simulink model "DPLL"  (R2013a)
settings: Solver=ode45  StartTime=0.0  StopTime=12000/1200  RelTol=1e-3
undefined symbols (not defined in the file): DiscIntNeverNeededParam
libraries: dspsigops x4, commfilt2 x3, dsparch4 x3, commsynccomp2 x2, commchan3 x1, commsink2 x1, commrandsrc2 x1
settings Model: Creator=Cedric  LastModifiedBy=Cedric

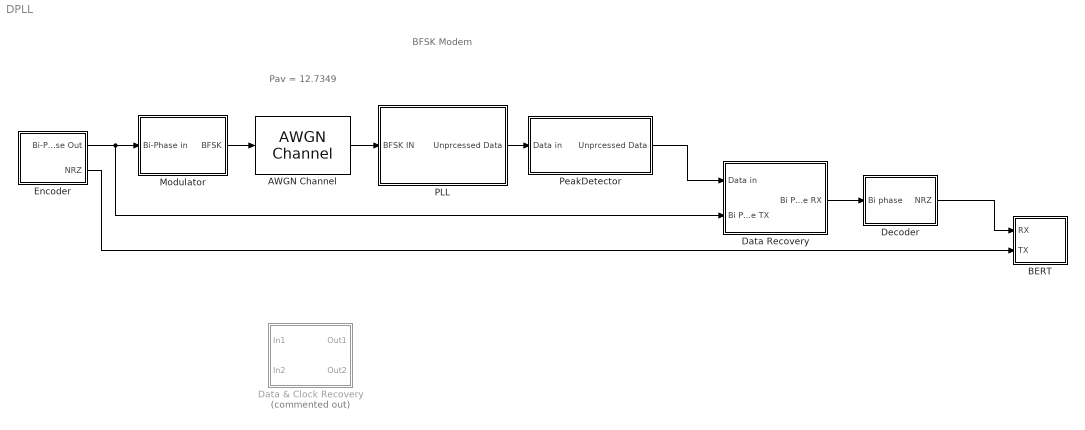
== system DPLL ==
  note: BFSK Modem
  note: Pav = 12.7349
  AWGN Channel : commchan3/AWGN Channel  InputProcessing=Columns as channels (frame based)  seed=randseed  noiseMode="Signal to noise ratio  (SNR)"  EbNodB=10  EsNodB=10  SNRdB=1000  bitsPerSym=1  Ps=12.7349  Tsym=1  variance=5
  BERT : Subsystem
  Data & Clock Recovery : Subsystem  Commented=on
  Data Recovery : Subsystem
  Decoder : Subsystem
  Encoder : Subsystem
  Modulator : Subsystem
  PLL : Subsystem
  PeakDetector : Subsystem
  wires:
  Modulator/1(BFSK) -> AWGN Channel/1
  Decoder/1(NRZ) -> BERT/1(RX)
  AWGN Channel/1 -> PLL/1(BFSK IN)
  Encoder/2(NRZ) -> BERT/2("TX ")
  PLL/1(Unprcessed Data) -> PeakDetector/1(Data in)
  Encoder/1(Bi-Phase Out) -> Data Recovery/2(Bi Phase TX), Modulator/1(Bi-Phase in)
  PeakDetector/1(Unprcessed Data) -> Data Recovery/1(Data in)
  Data Recovery/1(Bi Phase RX) -> Decoder/1(Bi phase)

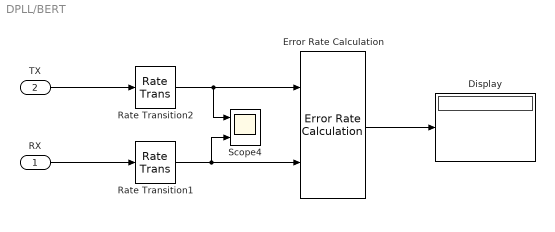
== system DPLL/BERT ==
  RX : Inport
  "TX " : Inport  Port=2
  Display : Display
  Error Rate Calculation : commsink2/Error Rate Calculation  N=1  st_delay=0  cp_mode=Entire frame  subframe=[]  PMode=Port  WsName=ErrorVec  RsMode2=off  stop=off  numErr=100  maxBits=1e6
  Rate Transition1 : RateTransition  OutPortSampleTime=1/(1200)
  Rate Transition2 : RateTransition  OutPortSampleTime=1/(1200)
  Scope4 : Scope  NumInputPorts=2
      settings: YMin=47500~-0.5  YMax=90000~1.5  SaveName=ScopeData3
  wires:
  Error Rate Calculation/1 -> Display/1
  "TX "/1 -> Rate Transition2/1
  RX/1 -> Rate Transition1/1
  Rate Transition1/1 -> Scope4/2, Error Rate Calculation/2
  Rate Transition2/1 -> Scope4/1, Error Rate Calculation/1

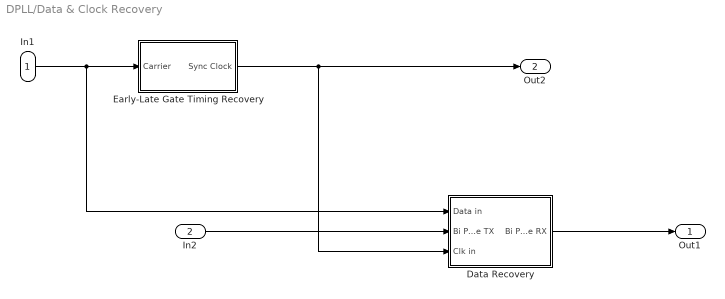
== system DPLL/Data & Clock Recovery ==
  In1 : Inport
  In2 : Inport  Port=2
  Data Recovery : Subsystem
  Early-Late Gate Timing Recovery : Subsystem
  Out1 : Outport
  Out2 : Outport  Port=2
  wires:
  Data Recovery/1(Bi Phase RX) -> Out1/1
  In2/1 -> Data Recovery/2(Bi Phase TX)
  Early-Late Gate Timing Recovery/1(Sync Clock) -> Data Recovery/3(Clk in), Out2/1
  In1/1 -> Early-Late Gate Timing Recovery/1(Carrier), Data Recovery/1(Data in)

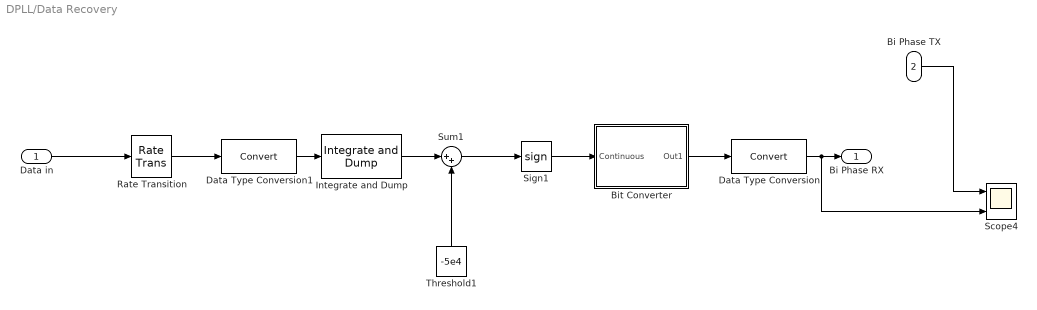
== system DPLL/Data Recovery ==
  Data in : Inport
  Bi Phase TX : Inport  Port=2
  Bit Converter : Subsystem
  Data Type Conversion : DataTypeConversion
  Data Type Conversion1 : DataTypeConversion
  Integrate and Dump : commfilt2/Integrate and Dump  obssamples=1024  offsetsamples=0  nodump=off  roundingMode=Floor  overflowMode=off
  Rate Transition : RateTransition  OutPortSampleTime=1/(1200*1024)
  Scope4 : Scope  NumInputPorts=2
      settings: YMin=47500~-0.5  YMax=90000~1.5  SaveName=ScopeData8
  Sign1 : Signum
  Sum1 : Sum  Inputs=|++
  Threshold1 : Constant  Value=-5e4
  Bi Phase RX : Outport
  wires:
  Data in/1 -> Rate Transition/1
  Bit Converter/1(Out1) -> Data Type Conversion/1
  Data Type Conversion/1 -> Scope4/2, Bi Phase RX/1
  Integrate and Dump/1 -> Sum1/1
  Data Type Conversion1/1 -> Integrate and Dump/1
  Rate Transition/1 -> Data Type Conversion1/1
  Threshold1/1 -> Sum1/2
  Sum1/1 -> Sign1/1
  Sign1/1 -> Bit Converter/1(Continuous)
  Bi Phase TX/1 -> Scope4/1

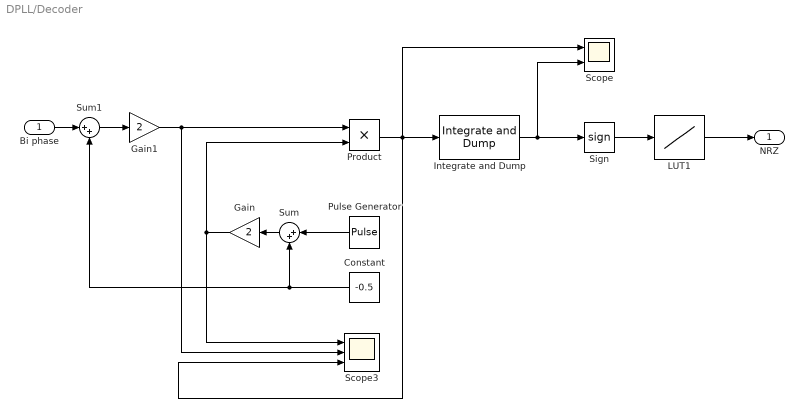
== system DPLL/Decoder ==
  Bi phase : Inport
  Constant : Constant  Value=-0.5
  Gain : Gain  Gain=2
  Gain1 : Gain  Gain=2
  Integrate and Dump : commfilt2/Integrate and Dump  obssamples=1024  offsetsamples=0  nodump=off  roundingMode=Floor  overflowMode=off
  LUT1 : Lookup_n-D  NumberOfTableDimensions=1  BreakpointsForDimension1=[-1 0 1]  Table=[0 0 1]  RndMeth=Simplest  InputSameDT=on
  Product : Product
  Pulse Generator : DiscretePulseGenerator  Period=2048*2  PulseWidth=2048  SampleTime=1/(1200*2048)
  Scope : Scope  NumInputPorts=2
      settings: YMin=-5~-5  YMax=5~5
  Scope3 : Scope  NumInputPorts=3
      settings: YMin=-1.5~-1.5~-1.5  YMax=1.5~1.5~1.5  SaveName=ScopeData5
  Sign : Signum
  Sum : Sum  Inputs=|++
  Sum1 : Sum  Inputs=|++
  NRZ : Outport
  wires:
  Integrate and Dump/1 -> Scope/2, Sign/1
  Product/1 -> Scope/1, Scope3/3, Integrate and Dump/1
  Pulse Generator/1 -> Sum/1
  Sum/1 -> Gain/1
  Constant/1 -> Sum1/2, Sum/2
  Gain/1 -> Product/2, Scope3/1
  Bi phase/1 -> Sum1/1
  Sum1/1 -> Gain1/1
  Gain1/1 -> Scope3/2, Product/1
  LUT1/1 -> NRZ/1
  Sign/1 -> LUT1/1

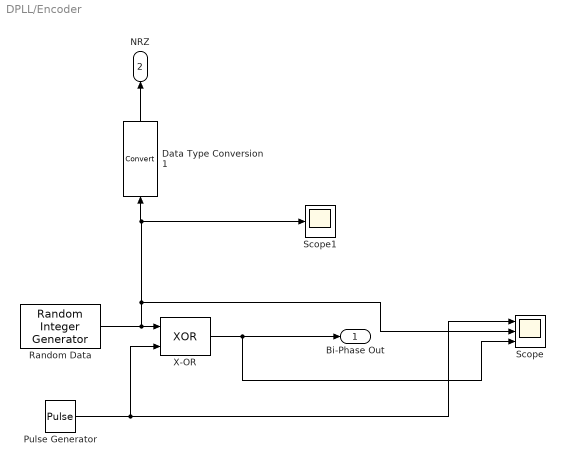
== system DPLL/Encoder ==
  Data Type Conversion1 : DataTypeConversion
  Pulse Generator : DiscretePulseGenerator  Period=2048*2  PulseWidth=2048  SampleTime=1/(1200*2048)
  Random Data : commrandsrc2/Random Integer Generator  mul=2  seed=randseed  Ts=1/600  frameBased=off  sampPerFrame=1  orient=off  outDataType=boolean
  Scope : Scope  NumInputPorts=3
      settings: TimeRange=0.007754789272030654  YMin=-0.5~-0.5~-0.5  YMax=1.5~1.5~1.5  SaveName=ScopeData7
  Scope1 : Scope
      settings: TimeRange=0.007754789272030654  YMin=-0.5  YMax=1.5  SaveName=ScopeData2
  X-OR : Logic  Operator=XOR  IconShape=distinctive  AllPortsSameDT=off  OutDataTypeStr=boolean
  Bi-Phase Out : Outport
  NRZ : Outport  Port=2
  wires:
  Random Data/1 -> Scope1/1, Data Type Conversion1/1, Scope/2, X-OR/1
  Pulse Generator/1 -> Scope/1, X-OR/2
  X-OR/1 -> Scope/3, Bi-Phase Out/1
  Data Type Conversion1/1 -> NRZ/1

== system DPLL/Modulator ==
  Bi-Phase in : Inport
  BFSK Modulator : Subsystem
  Scope : Scope
      settings: TimeRange=0.007754789272030654  YMin=0.06833333333333358  YMax=0.101666666666667  SaveName=ScopeData4
  BFSK : Outport
  wires:
  BFSK Modulator/1(BFSK out) -> Scope/1, BFSK/1
  Bi-Phase in/1 -> BFSK Modulator/1(Bi-phase L in)

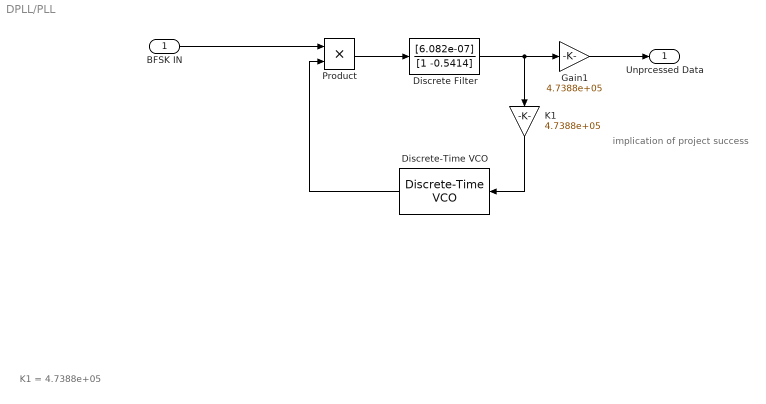
== system DPLL/PLL ==
  note: K1 = 4.7388e+05
  note: implication of project success
  BFSK IN : Inport
  Discrete Filter : DiscreteFilter  Numerator=[6.082e-07]  Denominator=[1 -0.5414]  SampleTime=1/(1200*1024)
  Discrete-Time VCO : commsynccomp2/Discrete-Time VCO  Ac=5  Fc=2200  Kc=1  Ph=0  ts=1/(1200*2048)
  Gain1 : Gain  Gain=4.7388e+05
  K1 : Gain  Gain=4.7388e+05
  Product : Product
  Unprcessed Data : Outport
  wires:
  Discrete-Time VCO/1 -> Product/2
  Product/1 -> Discrete Filter/1
  BFSK IN/1 -> Product/1
  Discrete Filter/1 -> K1/1, Gain1/1
  K1/1 -> Discrete-Time VCO/1
  Gain1/1 -> Unprcessed Data/1

== system DPLL/PeakDetector ==
  Data in : Inport
  Low Pass : dsparch4/Analog Filter Design  method=Butterworth  filttype=Lowpass  N=2  Wlo=2*pi*2400  Whi=80  Rp=2  Rs=40
  Product : Product
  Unprcessed Data : Outport
  wires:
  Data in/1 -> Product/2, Product/1
  Product/1 -> Low Pass/1
  Low Pass/1 -> Unprcessed Data/1

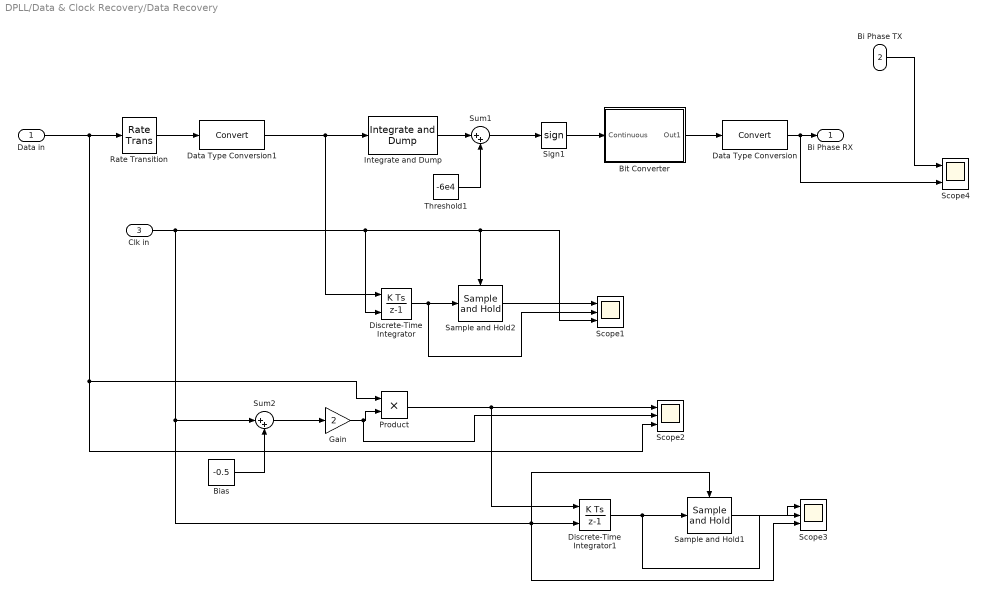
== system DPLL/Data & Clock Recovery/Data Recovery ==
  Data in : Inport
  Bi Phase TX : Inport  Port=2
  Clk in : Inport  Port=3
  Bias : Constant  Value=-0.5
  Bit Converter : Subsystem
  Data Type Conversion : DataTypeConversion
  Data Type Conversion1 : DataTypeConversion
  Discrete-Time Integrator : DiscreteIntegrator  ExternalReset=rising  SampleTime=1/(1200*1024)  ICPrevOutput=DiscIntNeverNeededParam  ICPrevScaledInput=DiscIntNeverNeededParam
  Discrete-Time Integrator1 : DiscreteIntegrator  ExternalReset=rising  SampleTime=1/(1200*1024)  ICPrevOutput=DiscIntNeverNeededParam  ICPrevScaledInput=DiscIntNeverNeededParam
  Gain : Gain  Gain=2
  Integrate and Dump : commfilt2/Integrate and Dump  obssamples=1024  offsetsamples=0  nodump=off  roundingMode=Floor  overflowMode=off
  Product : Product
  Rate Transition : RateTransition  OutPortSampleTime=1/(1200*1024)
  Sample and Hold1 : dspsigops/Sample and Hold  trig=Either edge  initCond=0  latchinput=off
  Sample and Hold2 : dspsigops/Sample and Hold  trig=Falling edge  initCond=0  latchinput=off
  Scope1 : Scope  NumInputPorts=3
      settings: YMin=0.005075~0~-5  YMax=0.00545~0.011~5  SaveName=ScopeData18
  Scope2 : Scope  NumInputPorts=3
      settings: YMin=-12.5~-1~2  YMax=12.5~1~13  SaveName=ScopeData19
  Scope3 : Scope  NumInputPorts=3
      settings: YMin=0~-0.003~-5  YMax=0.0065~0.007~5  SaveName=ScopeData20
  Scope4 : Scope  NumInputPorts=2
      settings: YMin=47500~-0.5  YMax=90000~1.5  SaveName=ScopeData8
  Sign1 : Signum
  Sum1 : Sum  Inputs=|++
  Sum2 : Sum  Inputs=|++
  Threshold1 : Constant  Value=-6e4
  Bi Phase RX : Outport
  wires:
  Data in/1 -> Scope2/3, Product/1, Rate Transition/1
  Bit Converter/1(Out1) -> Data Type Conversion/1
  Data Type Conversion/1 -> Scope4/2, Bi Phase RX/1
  Integrate and Dump/1 -> Sum1/1
  Data Type Conversion1/1 -> Discrete-Time Integrator/1, Integrate and Dump/1
  Rate Transition/1 -> Data Type Conversion1/1
  Threshold1/1 -> Sum1/2
  Sum1/1 -> Sign1/1
  Sign1/1 -> Bit Converter/1(Continuous)
  Bi Phase TX/1 -> Scope4/1
  Discrete-Time Integrator/1 -> Scope1/2, Sample and Hold2/1
  Clk in/1 -> Sum2/1, Scope3/3, Discrete-Time Integrator1/2, Sample and Hold1/Trigger, Scope1/3, Sample and Hold2/Trigger, Discrete-Time Integrator/2
  Sample and Hold2/1 -> Scope1/1
  Sum2/1 -> Gain/1
  Bias/1 -> Sum2/2
  Gain/1 -> Scope2/2, Product/2
  Product/1 -> Discrete-Time Integrator1/1, Scope2/1
  Discrete-Time Integrator1/1 -> Scope3/2, Sample and Hold1/1
  Sample and Hold1/1 -> Scope3/1

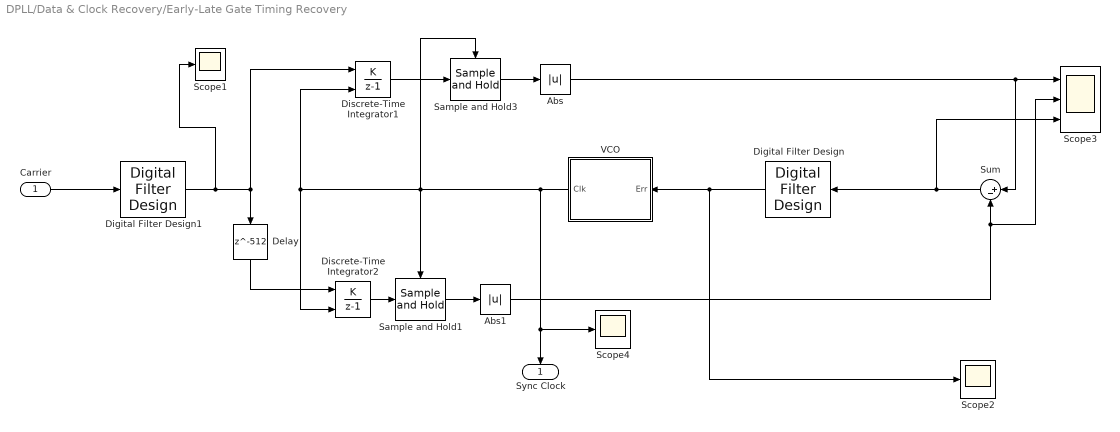
== system DPLL/Data & Clock Recovery/Early-Late Gate Timing Recovery ==
  Carrier : Inport
  Abs : Abs
  Abs1 : Abs
  Delay : Delay  DelayLength=512  InitialCondition=0  SampleTime=1/(1024*1200)
  Digital Filter Design : dsparch4/Digital Filter Design  mwdsp_browser_bugfix_var=off
  Digital Filter Design1 : dsparch4/Digital Filter Design  mwdsp_browser_bugfix_var=off
  Discrete-Time Integrator1 : DiscreteIntegrator  IntegratorMethod=Accumulation: Forward Euler  ExternalReset=rising  SampleTime=1/(1200*1024)  ICPrevOutput=DiscIntNeverNeededParam  ICPrevScaledInput=DiscIntNeverNeededParam
  Discrete-Time Integrator2 : DiscreteIntegrator  IntegratorMethod=Accumulation: Forward Euler  ExternalReset=rising  SampleTime=1/(1200*1024)  ICPrevOutput=DiscIntNeverNeededParam  ICPrevScaledInput=DiscIntNeverNeededParam
  Sample and Hold1 : dspsigops/Sample and Hold  trig=Either edge  initCond=0  latchinput=off
  Sample and Hold3 : dspsigops/Sample and Hold  trig=Either edge  initCond=0  latchinput=off
  Scope1 : Scope
      settings: YMin=-1  YMax=1  SaveName=ScopeData6
  Scope2 : Scope
      settings: YMin=-1  YMax=1  SaveName=ScopeData10
  Scope3 : Scope  NumInputPorts=3
      settings: YMin=-1~-5~-5  YMax=1~5~5  SaveName=ScopeData13
  Scope4 : Scope
      settings: YMin=-1  YMax=1  SaveName=ScopeData17
  Sum : Sum  Inputs=|+-
  VCO : Subsystem
  Sync Clock : Outport
  wires:
  Abs/1 -> Sum/1, Scope3/1
  Abs1/1 -> Scope3/2, Sum/2
  Delay/1 -> Discrete-Time Integrator2/1
  Discrete-Time Integrator1/1 -> Sample and Hold3/1
  Sample and Hold3/1 -> Abs/1
  Discrete-Time Integrator2/1 -> Sample and Hold1/1
  Sample and Hold1/1 -> Abs1/1
  Digital Filter Design/1 -> Scope2/1, VCO/1(Err)
  Carrier/1 -> Digital Filter Design1/1
  Sum/1 -> Scope3/3, Digital Filter Design/1
  Digital Filter Design1/1 -> Scope1/1, Delay/1, Discrete-Time Integrator1/1
  VCO/1(Clk) -> Sample and Hold3/Trigger, Discrete-Time Integrator1/2, Discrete-Time Integrator2/2, Sample and Hold1/Trigger, Scope4/1, Sync Clock/1

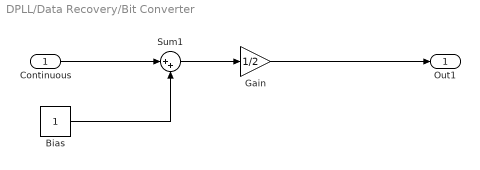
== system DPLL/Data Recovery/Bit Converter ==
  Continuous : Inport
  Bias : Constant
  Gain : Gain  Gain=1/2
  Sum1 : Sum  Inputs=|++
  Out1 : Outport
  wires:
  Gain/1 -> Out1/1
  Sum1/1 -> Gain/1
  Continuous/1 -> Sum1/1
  Bias/1 -> Sum1/2

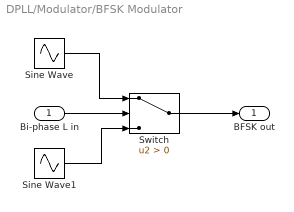
== system DPLL/Modulator/BFSK Modulator ==
  Bi-phase L in : Inport
  Sine Wave : Sin  SineType=Sample based  Amplitude=5  Frequency=2*pi*1200  Samples=2048  SampleTime=1/(1200*2048)
  Sine Wave1 : Sin  SineType=Sample based  Amplitude=5  Frequency=2*pi*2200  Samples=1117  SampleTime=1/(1200*2048)
  Switch : Switch  Criteria=u2 > Threshold  SampleTime=1/(1200*1024)
  BFSK out : Outport
  wires:
  Bi-phase L in/1 -> Switch/2
  Sine Wave/1 -> Switch/1
  Switch/1 -> BFSK out/1
  Sine Wave1/1 -> Switch/3

== system DPLL/Data & Clock Recovery/Data Recovery/Bit Converter ==
  Continuous : Inport
  Bias : Constant
  Gain : Gain  Gain=1/2
  Sum1 : Sum  Inputs=|++
  Out1 : Outport
  wires:
  Gain/1 -> Out1/1
  Sum1/1 -> Gain/1
  Continuous/1 -> Sum1/1
  Bias/1 -> Sum1/2

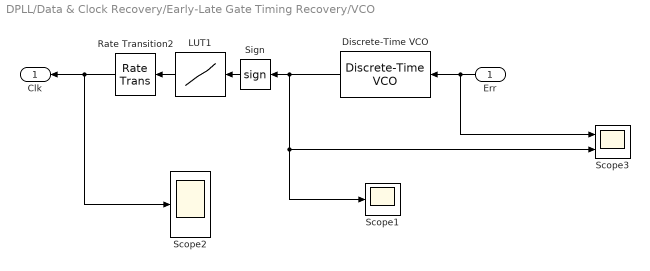
== system DPLL/Data & Clock Recovery/Early-Late Gate Timing Recovery/VCO ==
  Err : Inport
  Discrete-Time VCO : commsynccomp2/Discrete-Time VCO  Ac=1  Fc=600  Kc=0.125  Ph=0  ts=1/(1200*1024)
  LUT1 : Lookup_n-D  NumberOfTableDimensions=1  BreakpointsForDimension1=[-1 0 1]  Table=[0 0 1]  RndMeth=Simplest  InputSameDT=on
  Rate Transition2 : RateTransition  OutPortSampleTime=1/(1024*1200)
  Scope1 : Scope
      settings: TimeRange=0.01666666666666667  YMin=-1  YMax=1  SaveName=ScopeData15
  Scope2 : Scope
      settings: TimeRange=0.01666666666666667  YMin=-1  YMax=1  SaveName=ScopeData14
  Scope3 : Scope  NumInputPorts=2
      settings: TimeRange=0.01666666666666667  YMin=-1~-5  YMax=1~5  SaveName=ScopeData16
  Sign : Signum
  Clk : Outport
  wires:
  Discrete-Time VCO/1 -> Scope3/2, Scope1/1, Sign/1
  Err/1 -> Scope3/1, Discrete-Time VCO/1
  LUT1/1 -> Rate Transition2/1
  Rate Transition2/1 -> Scope2/1, Clk/1
  Sign/1 -> LUT1/1
